simulink model "RRR_PD_CT"  (R2022a)
settings: Solver=VariableStepAuto  StartTime=0.0  StopTime=150  RelTol=1e-6
undefined symbols (not defined in the file): controller, DiscIntNeverNeededParam, dq0, Kp_CT, Kp_PD, Kv_CT, Kv_PD, Levenberg, m1, m2, m3, Marquardt, p0, param, q0, r0, r1, r2, rel_err, slow
libraries: simulink x2, robotmaniplib x1
settings Model: PauseTimes=2.88  Creator=Mathew  LastModifiedBy=Marco
settings SolverCC: ZeroCrossControl=DisableAll  ODENIntegrationMethod=ode1be
settings DebuggingCC: AlgebraicLoopMsg=none  UnconnectedInputMsg=warning  UnconnectedOutputMsg=warning  UnconnectedLineMsg=warning  SFMachineParentedDataDiag=warning
settings SFSimCC: CustomCodeUndefinedFunction=UseInterfaceOnly
settings RTWCC: DLArmComputeVersion=19.05

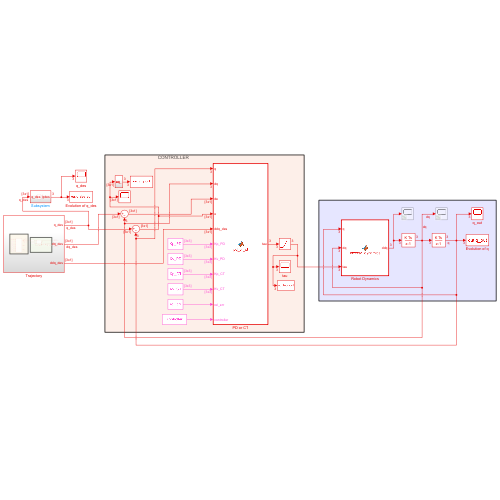
[thumbnail: Simulink's stored preview of the top-level diagram]
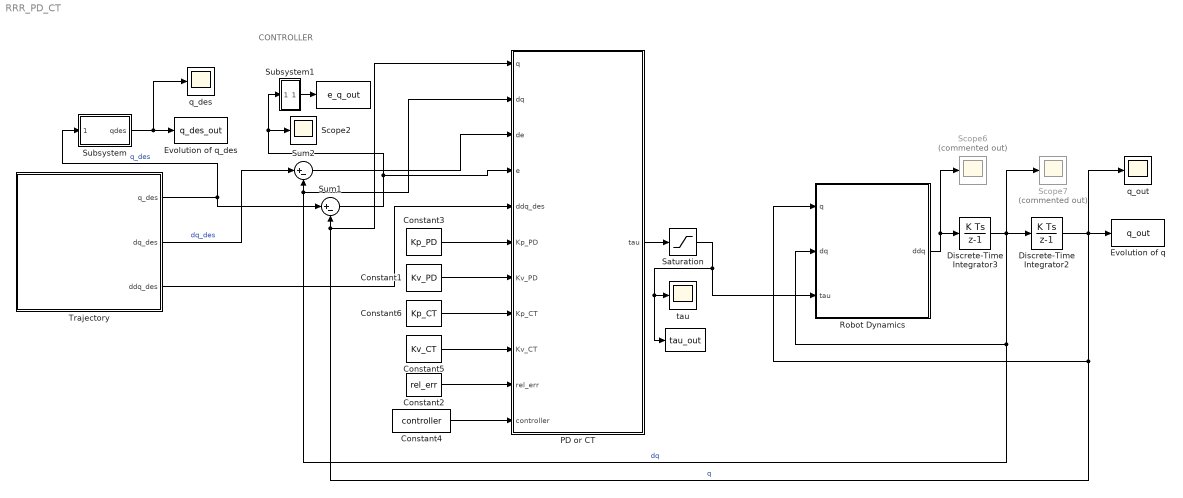
== system RRR_PD_CT ==
  note: CONTROLLER
  "   " : ToWorkspace  VariableName=e_q_out  SaveFormat=Timeseries  SampleTime=-1
  "         " : ToWorkspace  VariableName=tau_out  SaveFormat=Timeseries  SampleTime=-1
  Constant1 : Constant  Value=Kv_PD
  Constant2 : Constant  Value=rel_err
  Constant3 : Constant  Value=Kp_PD
  Constant4 : Constant  Value=controller
  Constant5 : Constant  Value=Kv_CT
  Constant6 : Constant  Value=Kp_CT
  Discrete-Time Integrator2 : DiscreteIntegrator  InitialCondition=q0  SampleTime=-1  ICPrevOutput=DiscIntNeverNeededParam  ICPrevScaledInput=DiscIntNeverNeededParam
  Discrete-Time Integrator3 : DiscreteIntegrator  InitialCondition=dq0  SampleTime=-1  ICPrevOutput=DiscIntNeverNeededParam  ICPrevScaledInput=DiscIntNeverNeededParam
  Evolution of q : ToWorkspace  VariableName=q_out  SaveFormat=Timeseries  SampleTime=-1
  Evolution of q_des : ToWorkspace  VariableName=q_des_out  SaveFormat=Timeseries  SampleTime=-1
  PD or CT : MATLAB Function  TreatAsAtomicUnit=on
  Robot Dynamics : MATLAB Function  TreatAsAtomicUnit=on
  Saturation : Saturate  UpperLimit=100  LowerLimit=-100
  Scope2 : Scope
  Scope6 : Scope  Commented=on
  Scope7 : Scope  Commented=on
  Subsystem : Subsystem
  Subsystem1 : Subsystem
  Sum1 : Sum  Inputs=|+-
  Sum2 : Sum  Inputs=|+-
  Trajectory : Subsystem
  q_des : Scope
  q_out : Scope
  tau : Scope
  wires:
  PD or CT/1(tau) -> Saturation/1
  Sum2/1 -> PD or CT/3(de)
  Constant2/1 -> PD or CT/10(rel_err)
  Constant3/1 -> PD or CT/6(Kp_PD)
  Constant1/1 -> PD or CT/7(Kv_PD)
  Sum1/1 -> Scope2/1, Subsystem1/1(eq), PD or CT/4(e)
  Constant4/1 -> PD or CT/11(controller)
  Constant6/1 -> PD or CT/8(Kp_CT)
  Constant5/1 -> PD or CT/9(Kv_CT)
  Subsystem/1(qdes) -> q_des/1, Evolution of q_des/1
  Trajectory/3(ddq_des) -> PD or CT/5(ddq_des)
  Trajectory/1(q_des) -> Sum1/1, Subsystem/1(q_des)  "q_des"
  Trajectory/2(dq_des) -> Sum2/1  "dq_des"
  Robot Dynamics/1(ddq) -> Discrete-Time Integrator3/1, Scope6/1
  Discrete-Time Integrator2/1 -> Robot Dynamics/1(q), PD or CT/1(q), Sum1/2, Evolution of q/1, q_out/1  "q"
  Discrete-Time Integrator3/1 -> Robot Dynamics/2(dq), PD or CT/2(dq), Sum2/2, Discrete-Time Integrator2/1, Scope7/1  "dq"
  Saturation/1 -> "         "/1, tau/1, Robot Dynamics/3(tau)
  Subsystem1/1(eq_) -> "   "/1

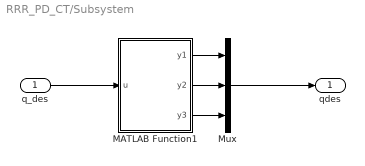
== system RRR_PD_CT/Subsystem ==
  q_des : Inport
  MATLAB Function1 : MATLAB Function  TreatAsAtomicUnit=on
  Mux : Mux  Inputs=3
  qdes : Outport
  wires:
  MATLAB Function1/1(y1) -> Mux/1
  Mux/1 -> qdes/1
  q_des/1 -> MATLAB Function1/1(u)
  MATLAB Function1/2(y2) -> Mux/2
  MATLAB Function1/3(y3) -> Mux/3

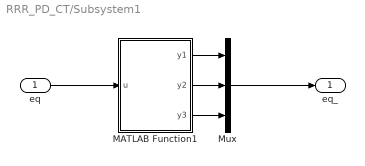
== system RRR_PD_CT/Subsystem1 ==
  eq : Inport
  MATLAB Function1 : MATLAB Function  TreatAsAtomicUnit=on
  Mux : Mux  Inputs=3
  eq_ : Outport
  wires:
  MATLAB Function1/3(y3) -> Mux/3
  MATLAB Function1/2(y2) -> Mux/2
  eq/1 -> MATLAB Function1/1(u)
  Mux/1 -> eq_/1
  MATLAB Function1/1(y1) -> Mux/1

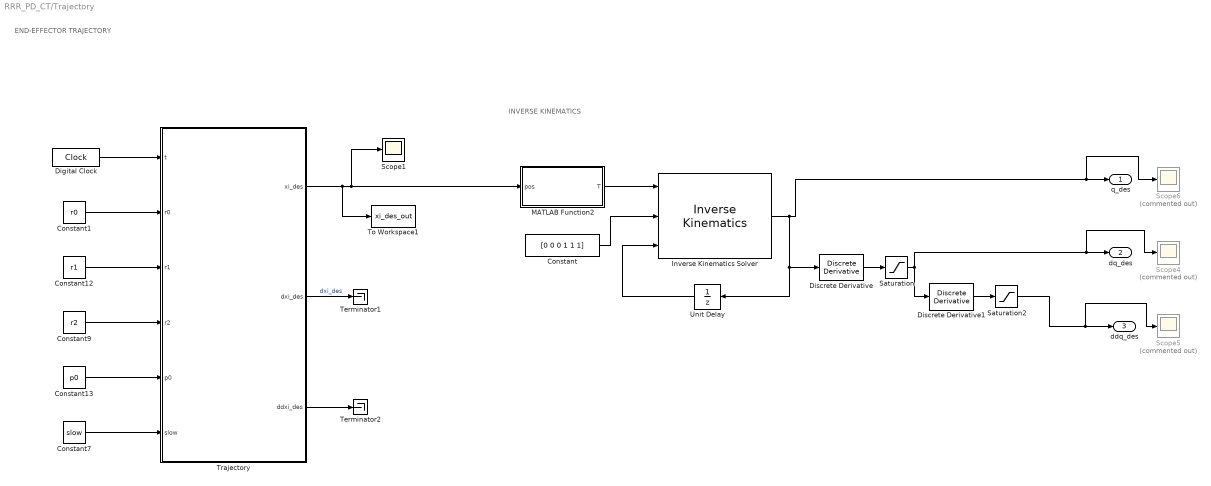
== system RRR_PD_CT/Trajectory ==
  note: END-EFFECTOR TRAJECTORY
  note: INVERSE KINEMATICS
  Constant : Constant  Value=[0 0 0 1 1 1]
  Constant1 : Constant  Value=r0
  Constant12 : Constant  Value=r1
  Constant13 : Constant  Value=p0
  Constant7 : Constant  Value=slow
  Constant9 : Constant  Value=r2
  Digital Clock : DigitalClock  SampleTime=0.01
  Discrete Derivative : simulink/Discrete/Discrete Derivative  gainval=1  ICPrevScaledInput=q0  OutMin=-1  OutMax=1  OutDataType=fixdt(1, 16)  OutScaling=2^-10  DoSatur=on
  Discrete Derivative1 : simulink/Discrete/Discrete Derivative  gainval=1.0  ICPrevScaledInput=ddq0  OutMin=[]  OutMax=[]  OutDataType=fixdt(1, 16)  OutScaling=2^-10  DoSatur=off
  Inverse Kinematics Solver : robotmaniplib/Inverse Kinematics  RigidBodyTree=ur10e_bis  EndEffector=body3  ShowInfo=off  SolverName=Levenberg-Marquardt  EnforceJointLimits=on  MaxIterations=1500  MaxTime=10  GradientTolerance=1e-7  SolutionTolerance=1e-5  StepTolerance=1e-14  ErrorChangeTolerance=1e-8  UseErrorDamping=on  DampingBias=0.0025  SimulateUsing=Interpreted execution
  MATLAB Function2 : MATLAB Function  TreatAsAtomicUnit=on
  Saturation : Saturate
  Saturation2 : Saturate  UpperLimit=0.1  LowerLimit=-0.1
  Scope1 : Scope
  Scope4 : Scope  Commented=on
  Scope5 : Scope  Commented=on
  Scope6 : Scope  Commented=on
  Terminator1 : Terminator
  Terminator2 : Terminator
  To Workspace1 : ToWorkspace  VariableName=xi_des_out  SaveFormat=Timeseries  SampleTime=-1
  Trajectory : MATLAB Function  TreatAsAtomicUnit=on
  Unit Delay : UnitDelay  SampleTime=-1  HasFrameUpgradeWarning=on
  q_des : Outport  VectorParamsAs1DForOutWhenUnconnected=off
  dq_des : Outport  Port=2  VectorParamsAs1DForOutWhenUnconnected=off
  ddq_des : Outport  Port=3  VectorParamsAs1DForOutWhenUnconnected=off
  wires:
  Trajectory/1(xi_des) -> Scope1/1, MATLAB Function2/1(pos), To Workspace1/1
  Constant13/1 -> Trajectory/5(p0)
  Constant7/1 -> Trajectory/6(slow)
  Constant9/1 -> Trajectory/4(r2)
  Constant12/1 -> Trajectory/3(r1)
  Trajectory/3(ddxi_des) -> Terminator2/1
  Inverse Kinematics Solver/1 -> Unit Delay/1, Discrete Derivative/1, Scope6/1, q_des/1
  Constant/1 -> Inverse Kinematics Solver/2
  MATLAB Function2/1(T) -> Inverse Kinematics Solver/1
  Unit Delay/1 -> Inverse Kinematics Solver/3
  Digital Clock/1 -> Trajectory/1(t)
  Trajectory/2(dxi_des) -> Terminator1/1  "dxi_des"
  Discrete Derivative/1 -> Saturation/1
  Discrete Derivative1/1 -> Saturation2/1
  Saturation/1 -> Discrete Derivative1/1, Scope4/1, dq_des/1
  Saturation2/1 -> Scope5/1, ddq_des/1
  Constant1/1 -> Trajectory/2(r0)

== matlab function RRR_PD_CT/Subsystem1/MATLAB Function1 ==
  data: u input; y1 output; y2 output; y3 output
function [y1,y2,y3] = fcn(u)

y1 = squeeze(u(1));
y2 = squeeze(u(2));
y3 = squeeze(u(3));

== matlab function RRR_PD_CT/Subsystem/MATLAB Function1 ==
  data: u input; y1 output; y2 output; y3 output
function [y1,y2,y3] = fcn(u)

y1 = squeeze(u(1));
y2 = squeeze(u(2));
y3 = squeeze(u(3));

== matlab function RRR_PD_CT/Trajectory/Trajectory ==
  data: t input; r0 input; xi_des output; r1 input; r2 input; p0 input; slow input; dxi_des output; ddxi_des output
function [xi_des, dxi_des, ddxi_des] = trajectory(t,r0,r1,r2,p0,slow)

    k=slow;
    
    xi_des =   [r0*sin(t/(2*k))       ; r1*sin(t/k)     ; r2*cos(t/k)     ] + p0;
    dxi_des =  [r0/2/k*cos(t/(2*k))   ; r1/k*cos(t/k)   ; -r2/k*sin(t/k)  ];
    ddxi_des = [-r0/4/k/k*sin(t/(2*k)); -r1/k/k*sin(t/k); -r2/k/k*cos(t/k)];

end

== matlab function RRR_PD_CT/PD or CT ==
  data: q input; dq input; de input; e input; ddq_des input; tau output; Kp_PD input; Kv_PD input; Kp_CT input; Kv_CT input; rel_err input; controller input; m1 parameter; m2 parameter; m3 parameter; param parameter
function tau  = pd_or_ct(q, dq, de, e, ddq_des, Kp_PD, Kv_PD, Kp_CT, Kv_CT, rel_err,controller, m1, m2, m3,param)
  
    % Get gravity vector
    g = 9.81;
    
    % Get dynamic matrices
    M = B_3r(param,m1,m2,m3,q);
    C = C_3r(param,m1,m2,m3,q,dq);
    G = G_3r(g,param,m1,m2,m3,q);
    
    % Adding uncertainty
    M = M.*(1 + rel_err);
    C = C.*(1 + rel_err);
    G = G.*(1 + rel_err);
    
    if controller == 1
        % PD law
        tau = Kv_PD*de + Kp_PD*e + G;
    else
        % Computed_torque law
        tau = M*(ddq_des + Kv_CT*de + Kp_CT*e) + C*dq + G;
    end

end

== matlab function RRR_PD_CT/Trajectory/MATLAB Function2 ==
  data: pos input; T output
function T = homogeneus_transf(pos)
    
    T=eye(4);
    
    T = [  eye(3),     [pos(1);pos(2);pos(3) ];
         0 0 0              1           ]; 

end

== matlab function RRR_PD_CT/Robot Dynamics ==
  data: q input; dq input; tau input; ddq output; m1 parameter; m2 parameter; m3 parameter; param parameter
function ddq = inverse_dynamics(q, dq, tau,m1, m2, m3, param)
   
    g = 9.81;
    
    % Get dynamic matrices
    M = B_3r(param,m1,m2,m3,q);
    C = C_3r(param,m1,m2,m3,q,dq);
    G = G_3r(g,param,m1,m2,m3,q);
    
    ddq = pinv(M)*(tau - C*dq - G);

end
